simulink model "testemplanner_cs_old"  (R2020a)
settings: Solver=ode5  StartTime=0.0  StopTime=120  FixedStep=1/1000  RelTol=1e-3
PreLoadFcn:
  | mbxruntime.callbacks.PreLoadFcn(bdroot);
PostLoadFcn:
  | mbxruntime.callbacks.PostLoadFcn(bdroot);
InitFcn:
  | mbxruntime.callbacks.InitFcn(bdroot);
StartFcn:
  | mbxruntime.callbacks.StartFcn(bdroot);
StopFcn:
  | mbxruntime.callbacks.StopFcn(bdroot);
model workspace (MAT data in the model file):
  mbox_table : object (value not decoded)
  model_closed = 0
  sim_status = 0
values from neighbouring files (symbols this model uses):
  c_factor = 43.75    [emplanner_init.m]
  cf = -175016    [emplanner_init.m]
  cr = -130634    [emplanner_init.m]
  global_path_x = [0.057304 1.05668625507 2.05480936558 3.05165624935 4.04722112279 5.04150235808 6.03449985569 7.02621407764 8.01664569183 9.00579544113 9.99366409523 10.9802524329 ... (3001 elements, 3001x1)]    [global_path.mat]
  global_path_y = [8.29 8.29 8.29 8.29 8.29 8.29 8.29 8.29 8.29 8.29 8.29 8.29 ... (3001 elements, 3001x1)]    [global_path.mat]
  KD_PID_distance = 0.0    (= 0)    [emplanner_init.m]
  KD_PID_speed = 0    [emplanner_init.m]
  KI_PID_distance = 0.0    (= 0)    [emplanner_init.m]
  KI_PID_speed = 0    [emplanner_init.m]
  KP_PID_distance = 0.5    [emplanner_init.m]
  KP_PID_speed = 1.8    [emplanner_init.m]
  la = 1.265    [emplanner_init.m]
  lb = 2.947-1.265    (= 1.682)    [emplanner_init.m]
  LQR_K1 = k(:,1)'    [emplanner_init.m]
  LQR_K2 = k(:,2)'    [emplanner_init.m]
  LQR_K3 = k(:,3)'    [emplanner_init.m]
  LQR_K4 = k(:,4)'    [emplanner_init.m]
  m = 2020    [emplanner_init.m]
  rack_displacement = [-39.14 , -37.2 , -35.29 , -33.43 , -31.6 , -29.81 , -28.06 , -26.34 , -24.66 ,      -23.01 , -21.38 , -19.79 , -18.23 , -16.69 , -15.18 , -13.7 , -12.23 , -10.8 , -9.38 , -7.98 ,     -6.61 , -5.25 , -3.91 , -2.59 , -1.29 , 0 , 1.27 , 2.54 , 3.78 , 5.02 , 6.24 , 7.46 , 8.66 ,      9.86 , 11.05 , 12.24 , 13.41 , 14.59 , 15.76 , 16.92 , 18.09 , 19.25 , 20.42 , 21.59 , 22.76 ,      23.93 , 25.11 , 26 ...(+26 chars)    [emplanner_init.m]
  right_wheel_ground = [-70 ,-67.2 , -64.4 , -61.6 , -58.8 , -56 , -53.2 , -50.4 , -47.6 , -44.8 , -42 ,      -39.2 , -36.4 , -33.6 , -30.8 , -28 , -25.2 , -22.4 , -19.6 , -16.8 , -14 , -11.2 , -8.4 , -5.6 ,      -2.8 , 0 , 2.8 , 5.6 , 8.4 , 11.2 , 14 , 16.8 , 19.6 , 22.4 , 25.2 , 28 , 30.8 , 33.6 , 36.4 ,      39.2 , 42 , 44.8 , 47.6 , 50.4 , 53.2 , 56 , 58.8 , 61.6 , 64.4 , 67.2 , 70 ]    [emplanner_init.m]
  vx_break_point = zeros(1,5000)    [emplanner_init.m]
undefined symbols (not defined in the file or in its folder): aubr, DiscIntNeverNeededParam, tablebr, vubr
libraries: PreScanSimulinkLibrary x9, Solver_SF x1, simulink_extras x1
(part 5 of 6)

== matlab function testemplanner_cs_old/Audi_A8_Sedan_1/decision&planning module/EM_planner/calc plan start and stitch trajectory ==
  data: host_x input; plan_start_x output; host_y input; host_heading_xy input; host_vx input; host_vy input; host_ax input; host_ay input; pre_trajectory_x input; pre_trajectory_y input; pre_trajectory_heading input; pre_trajectory_kappa input; pre_trajectory_velocity input; pre_trajectory_accelerate input; pre_trajectory_time input; current_time input; plan_start_y output; plan_start_heading output; plan_start_kappa output; plan_start_vx output; plan_start_vy output; plan_start_ax output; plan_start_ay output; plan_start_time output; stitch_x output; stitch_y output; stitch_heading output; stitch_kappa output; stitch_velocity output; stitch_accelerate output; stitch_time output
function [plan_start_x,plan_start_y,plan_start_heading,plan_start_kappa,plan_start_vx,plan_start_vy,plan_start_ax,plan_start_ay,plan_start_time,stitch_x,stitch_y,...
    stitch_heading,stitch_kappa,stitch_velocity,stitch_accelerate,stitch_time] = fcn(host_x,host_y,host_heading_xy,host_vx,host_vy,host_ax,host_ay,pre_trajectory_x,pre_trajectory_y,...
    pre_trajectory_heading,pre_trajectory_kappa,pre_trajectory_velocity,pre_trajectory_accelerate,pre_trajectory_time,current_time)

%%作用：求得当前周期的规划起点，有两种方式，①一种方式是车辆当前位置与上一周期规划路径点相差较大，此时需要通过车辆动力学外推得到，②另一种方式是相差不大，直径将原有路径延长得到
%%输入：上一个周期规划出的路径的坐标点，航向，速度，加速度。车辆当前的坐标点、航向，速度，加速度，当前时间。
%%输出；规划起点的坐标点，航向，速度，加速度；待拼接轨迹的坐标点，航向，速度，加速度以及时间。

% 初始化待拼接轨迹，此轨迹主要用来进行拼接，加速计算过程，待拼接轨迹为计算的规划起点在原有轨迹上的位置向前取20个点，因此初始化一个20个点的数组
stitch_x=zeros(20,1)*nan;
stitch_y=zeros(20,1)*nan;
stitch_heading=zeros(20,1)*nan;
stitch_kappa=zeros(20,1)*nan;
stitch_velocity=zeros(20,1)*nan;
stitch_accelerate=zeros(20,1)*nan;
%时间初始化为-1，代表没有要拼接的轨迹
stitch_time=ones(20,1)*(-1);

%根据是否为第一次运行进行区分，
persistent is_first_run

if isempty(is_first_run)
    %算法首次运行，本来需要外推，但因为是首次运行就以车辆当前的位置作为规划起点
    is_first_run=0;
    plan_start_x=host_x;
    plan_start_y=host_y;
    plan_start_heading=host_heading_xy;
    plan_start_kappa=0;
    plan_start_vx=0;
    plan_start_vy=0;
    plan_start_ax=0;
    plan_start_ay=0;
    %规划起点时间戳为当前时间+100ms
    plan_start_time=current_time+0.1;
else
    %算法不是首次运行，可以正常运行
    
    %比较车辆当前实际位置与车辆规划位置的差别
    
    x_current=host_x;
    y_current=host_y;
    heading_current=host_heading_xy;
    kappa_current=0;%默认起点曲率为0
    %要转换为世界坐标系
    vx_current=host_vx*cos(heading_current)-host_vy*sin(heading_current);
    vy_current=host_vx*sin(heading_current)+host_vy*cos(heading_current);
    ax_current=host_ax*cos(heading_current)-host_ay*sin(heading_current);
    ay_current=host_ax*sin(heading_current)+host_ay*cos(heading_current);
    %接着遍历数组，求解根据规划，车辆当前应道在的位置
    for i=1:length(pre_trajectory_time)
        if(pre_trajectory_time(i)<=current_time)&&(pre_trajectory_time(i+1)>current_time)
           break; 
        else
        end
    end
    x_desire=pre_trajectory_x(i);
    y_desire=pre_trajectory_x(i);
    heading_desire=pre_trajectory_heading(i);
%     vx_desire=pre_trajectory_velocity*cos(pre_trajectory_heading(i));
%     vy_desire=pre_trajectory_velocity*sin(pre_trajectory_heading(i));
%     ax_desire=pre_trajectory_accelerate*cos(pre_trajectory_heading(i));
%     ay_desire=pre_trajectory_accelerate*sin(pre_trajectory_heading(i));
    
   %得到两个位置的误差
   %通过向量法计算误差
   %切向向量
   tor = [cos(heading_desire);sin(heading_desire)];
   %法向向量
   nor = [-sin(heading_desire);cos(heading_desire)];
   %两点向量
   error = [host_x;host_y]-[x_desire;y_desire];
   %纵向误差
   long_error = abs(error'*tor);
   %横向误差
   lat_error = abs(error'*nor);
   
   if (long_error>2.5)||(lat_error>0.5)   %控制误差过大，使用车辆动力学外推
        dt=0.1;
        plan_start_x=x_current+vx_current*dt+0.5*ax_current*dt*dt;
        plan_start_y=y_current+vy_current*dt+0.5*ay_current*dt*dt;
        plan_start_kappa=kappa_current;
        plan_start_vx=vx_current+ax_current*dt;
        plan_start_vy=vy_current+ay_current*dt;
        plan_start_ax=ax_current;
        plan_start_ay=ax_current;
        plan_start_heading=atan2(plan_start_vy,plan_start_vx);
    %规划起点时间戳为当前时间+100ms
        plan_start_time=current_time+0.1;
   else     %控制误差不大，则利用上一个周期规划路径找点
       for j=i:length(pre_trajectory_time)
            if (pre_trajectory_time(j)<=current_time+0.1)&&(pre_trajectory_time(j+1)>current_time+0.1)
                break;
            end
       end
        plan_start_x=pre_trajectory_x(j);
        plan_start_y=pre_trajectory_y(j);
        plan_start_heading=pre_trajectory_heading(j);
        plan_start_kappa=pre_trajectory_kappa(j);
        plan_start_vx=pre_trajectory_velocity(j)*cos(pre_trajectory_heading(j));
        plan_start_vy=pre_trajectory_velocity(j)*sin(pre_trajectory_heading(j));
        % 注意，由于是做圆周运动，所以加速度要先按照切向和法相进行分解
         %切向向量
         tor = [cos(heading_desire);sin(heading_desire)];
         %法向向量
         nor = [-sin(heading_desire);cos(heading_desire)];
        tor_a=pre_trajectory_accelerate(j)*tor;        %切向加速度
        nor_a=pre_trajectory_velocity(j)*pre_trajectory_kappa(j)*nor; %法向加速度=v^2/r
        %分别将切向加速度和法向加速度的x，y分量相加就是ax和ay
        plan_start_ax=tor_a(1)+nor_a(1);
        plan_start_ay=tor_a(2)+nor_a(2);
    %规划起点时间戳为当前时间+100ms
        plan_start_time=pre_trajectory_time(j); 
         %下面开始进行轨迹拼接
         %当前节点是j，如果j大于20，则往前拼接20个点，如果j<20，则能拼几个点就拼几个点。从stitch最后一个点开始拼，没有拼上的点time为-1
         if j>=21
             for k=j-1:-1:j-20
                 stitch_time(k)=pre_trajectory_time(k);
                 stitch_x(k)=pre_trajectory_x(k);
                 stitch_y(k)=pre_trajectory_y(k);
                 stitch_heading(k)=pre_trajectory_heading(k);
                 stitch_kappa(k)=pre_trajectory_kappa(k);
                 stitch_velocity(k) = pre_trajectory_velocity(k);
                 stitch_accelerate (k)= pre_trajectory_accelerate (k);
             end
         else
             for k=1:j-1
                 stitch_time(20+1-k)=pre_trajectory_time(j-k);
                 stitch_x(20+1-k)=pre_trajectory_x(j-k);
                 stitch_y(20+1-k)=pre_trajectory_y(j-k);
                 stitch_heading(20+1-k)=pre_trajectory_heading(j-k);
                 stitch_kappa(20+1-k)=pre_trajectory_kappa(j-k);
                 stitch_velocity(20+1-k) = pre_trajectory_velocity(j-k);
                 stitch_accelerate(20+1-k) = pre_trajectory_accelerate(j-k);
             end
         end
   end
   
   
   
end

== matlab function testemplanner_cs_old/Audi_A8_Sedan_1/decision&planning module/EM_planner/obs/Cart2Frenet/CalcSL2 ==
  data: frenet_l_set input; ax_set input; ay_set input; s_dot_set input; dl_set input; plan_start_proj_heading input; plan_start_proj_kappa input; s_dot2_set output; l_dot2_set output; ddl_set output
function [ s_dot2_set, l_dot2_set,ddl_set]=fcn(frenet_l_set,ax_set,ay_set,s_dot_set,dl_set,plan_start_proj_heading,plan_start_proj_kappa)
%作用：通过之前计算得到的l，s_dot、dl值以及已知的ax，ay值，计算s_dot2,l_dot2,以及ddl
 %首先做一个缓冲
 n=128;
 s_dot2_set=ones(n,1)*nan;
 l_dot2_set=ones(n,1)*nan;
 ddl_set=ones(n,1)*nan;

 for i=1:length(frenet_l_set)
     if isnan(frenet_l_set(i))
         break;
     end
    %先求自然坐标系的切向量和法向量
%切向量
tor=[cos(plan_start_proj_heading(i));sin(plan_start_proj_heading(i))];
%法向量
nor=[-sin(plan_start_proj_heading(i));cos(plan_start_proj_heading(i))];

ah=[ax_set(i);ay_set(i)];
l_dot2_set(i)=ah'*nor- plan_start_proj_kappa(i) * (1 - plan_start_proj_kappa(i) * frenet_l_set(i)) * s_dot_set(i)^2;
s_dot2_set(i)=(1/(1 - plan_start_proj_kappa(i) * frenet_l_set(i)))* (ah' * tor + 2 * plan_start_proj_kappa(i) * dl_set(i) * s_dot_set(i)^2);

if abs(s_dot2_set(i))<1e-6
    ddl_set(i)=0;
else
    ddl_set(i)=(l_dot2_set(i) - dl_set(i)*s_dot2_set(i))/(s_dot_set(i)^2);
 end
end

== matlab function testemplanner_cs_old/Audi_A8_Sedan_1/decision&planning module/EM_planner/obs/Cart2Frenet/Calcs_l_dot_dl ==
  data: frenet_l_set input; vx_set input; vy_set input; plan_start_proj_heading input; plan_start_proj_kappa input; s_dot_set output; l_dot_set output; dl_set output
function [ s_dot_set, l_dot_set,dl_set]=fcn(frenet_l_set,vx_set,vy_set,plan_start_proj_heading,plan_start_proj_kappa)
%作用：通过之前计算得到的s和l值以及计算的速度值，计算s_dot,l_dot,以及dl
 %首先做一个缓冲
 n=128;
 s_dot_set=ones(n,1)*nan;
 l_dot_set=ones(n,1)*nan;
 dl_set=ones(n,1)*nan;

 for i=1:length(frenet_l_set)
     if isnan(frenet_l_set(i))
         break;
     end
    %先求自然坐标系的切向量和法向量
%切向量
tor=[cos(plan_start_proj_heading(i));sin(plan_start_proj_heading(i))];
%法向量
nor=[-sin(plan_start_proj_heading(i));cos(plan_start_proj_heading(i))];

vh=[vx_set(i);vy_set(i)];
l_dot_set(i)=vh'*nor;
s_dot_set(i)=vh'*tor/(1-plan_start_proj_kappa(i)*frenet_l_set(i));

if abs(s_dot_set(i))<1e-6
    dl_set(i)=0;
else
    dl_set(i)=l_dot_set(i)/s_dot_set(i);
 end
end

== matlab function testemplanner_cs_old/Audi_A8_Sedan_1/decision&planning module/EM_planner/DP path ==
  data: plan_start_s input; dp_path_s_init output; plan_start_l input; plan_start_dl input; plan_start_ddl input; obs_s_set input; obs_l_set input; w_smooth_dl_cost input; w_collision_cost input; w_ref_cost input; w_smooth_ddl_cost input; w_smooth_dddl_cost input; col input; row input; sample_s input; sample_l input; dp_path_l_init output
function [dp_path_s_init,dp_path_l_init] = fcn(plan_start_s,plan_start_l,plan_start_dl,plan_start_ddl,obs_s_set,obs_l_set,w_smooth_dl_cost,w_collision_cost,w_ref_cost,w_smooth_ddl_cost,w_smooth_dddl_cost,col,row,sample_s,sample_l)
%%作用：撒点，通过动态规划算出代价最小的路径点集合，算出要进行优化的凸空间
%%输入：规划起点的s，l,dl,ddl,静态障碍物的s，l集合，dl，ddl，dddl平滑代价，参考线代价以及碰撞代价权重
%%行数：为奇数，列数；采样的横向距离以及纵向距离

%%输出：计算得到的路径点s，l初始值

%首先定义一个代价数组，代表从起点到当前i，j点的总代价，均初始化为inf无穷大
node=ones(col,row)*inf;

%再定义一个pre_node,用来表征node的父节点的坐标索引，均初始化为0，0；假设所有节点的父节点均为起点

pre_node=zeros(col,row);
%首先计算第一列的点的cost，调用CalccostFromStart函数进行计算
for i=1:row
    node(1,i)=CalccostFromStart(plan_start_s,plan_start_l,plan_start_dl,plan_start_ddl,obs_s_set,obs_l_set,w_smooth_dl_cost,w_collision_cost,w_ref_cost,w_smooth_ddl_cost,w_smooth_dddl_cost,i,row,sample_s,sample_l);
end
%计算从第二列开始的每一列的最小代价值以及其父节点的索引值，调用CalccostFromNeibor函数进行计算
for j=2:col
    for k =1:row
    [node,pre_node]=CalccostFromNeibor(plan_start_s,node,pre_node,k,j,obs_s_set,obs_l_set,w_smooth_dl_cost,w_collision_cost,w_ref_cost,w_smooth_ddl_cost,w_smooth_dddl_cost,row,sample_s,sample_l);
    end
end
% 找到最后一列中代价最小的节点
min_cost=node(1,end);
index=1;
for i=2:row
    min_cost_temp=node(i,end);
    if min_cost_temp<min_cost
        index=i;
        min_cost=min_cost_temp;
    else
    end
end

%因为不知道有多少个点，所以做一个缓冲
dp_path_s_init=ones(15,1)* -1;
dp_path_l_init=ones(15,1)* -1;

temp_node=zeros(15,1);

%从最后一个节点开始，反向找到最小代价路径上的所有点，并放入集合中
for i=col:-1:1
    
    temp_node(i)=pre_node(index,i);
    index=pre_node(index,i);
end
%确定路径上点的s，l值
for i=1:col
dp_path_s_init(i)=sample_s*i;
dp_path_l_init(i)=sample_l*(temp_node(col+1-i)-(row+1)/2);
end
end

%函数CalccostFromNeibor，计算从上一列的临近点到这个点的最小cost值和其父节点的行索引
function [node,pre_node]=CalccostFromNeibor(plan_start_s,node,pre_node,k,j,obs_s_set,obs_l_set,w_smooth_dl_cost,w_collision_cost,w_ref_cost,w_smooth_ddl_cost,w_smooth_dddl_cost,row,sample_s,sample_l)
% %作用： 计算从从上一列的临近点到这个点的最小cost值和其父节点的行索引
  %输入：起点的s，l，障碍物的s,l,dl,ddl,dddl平滑权重，障碍物碰撞权重，参考线权重，当前所在行数，列数，总行数，采样s，l，node和pre_node数组
  %输出：更新后的node和pre_node数组
  %dl，ddl设为0，因为DP仅仅是为了粗略开辟凸空间，不用太精细。
start_s=plan_start_s+sample_s*(j-1);
end_s=start_s+plan_start_s+sample_s*(j);
start_dl=0;
start_ddl=0;
end_dl=0;
end_ddl=0;
cost=zeros(row,1);
%确定起点和终点参数，计算五次多项式系数
for i=1:row
start_l=sample_l*(i-(row+1)/2);
end_l=sample_l*(k-(row+1)/2);
%调用函数计算五次多项式系数
coffee=Calccoffee(start_s,start_l,start_dl,start_ddl,end_s,end_l,end_dl,end_ddl);

s_set=zeros(10,1);
l_set=zeros(10,1);
dl_set=zeros(10,1);
ddl_set=zeros(10,1);
dddl_set=zeros(10,1);

%找10个点进行代价计算
for n=1:10
    s_set(n)=start_s+sample_s/10*(n-1);
    l_set(n)=coffee(1)*(s_set(n))^5+coffee(2)*(s_set(n))^4+coffee(3)*(s_set(n))^3+coffee(4)*(s_set(n))^2+coffee(5)*(s_set(n))+coffee(6);
    dl_set(n)=5*coffee(1)*(s_set(n))^4+4*coffee(2)*(s_set(n))^3+3*coffee(3)*(s_set(n))^2+2*coffee(4)*(s_set(n))+coffee(5);
    ddl_set(n)=20*coffee(1)*(s_set(n))^3+12*coffee(2)*(s_set(n))^2+6*coffee(3)*(s_set(n))+2*coffee(4);
    dddl_set(n)=60*coffee(1)*(s_set(n))^2+24*coffee(2)*(s_set(n))+6*coffee(3);
end
%首先计算平滑带代价和参考线代价
smooth_cost=w_smooth_dl_cost*(dl_set'*dl_set)+w_smooth_ddl_cost*(ddl_set'*ddl_set)+w_smooth_dddl_cost*(dddl_set'*dddl_set);
ref_cost=w_ref_cost*(l_set'*l_set);
%接着计算障碍物代价
collision_cost=0;
for m=1:length(obs_s_set)
    if isnan(obs_s_set(m))
        break;
    end
    s_err=obs_s_set(m)*ones(10,1)-s_set;
    l_err=obs_l_set(m)*ones(10,1)-l_set;
    err_squard=s_err.^2+l_err.^2;
    %调用障碍物代价模型函数CalcObsCost进行计算
    collision_cost_one=CalcObsCost(err_squard,w_collision_cost);
    collision_cost=collision_cost+collision_cost_one;
end

cost(i)=smooth_cost+ref_cost+collision_cost+node(i,j-1);
end
index=1;
min_cost=cost(1);
for h =2:row
   
    min_cost_temp=cost(h);
    if min_cost_temp<min_cost
        index=h;
        min_cost=min_cost_temp;
    else
    end
end
 pre_node(k,j)=index;
 node(k,j)=min_cost;
end




%函数CalccostFromStart，计算从起点到第一列的点的cost值
function cost=CalccostFromStart(plan_start_s,plan_start_l,plan_start_dl,plan_start_ddl,obs_s_set,obs_l_set,w_smooth_dl_cost,w_collision_cost,w_ref_cost,w_smooth_ddl_cost,w_smooth_dddl_cost,node_row,row,sample_s,sample_l)

  %作用： 计算从起点到第一列的点的cost值
  %输入：起点的s，l，dl，ddl,障碍物的s,l,dl,ddl,dddl平滑权重，障碍物碰撞权重，参考线权重，当前所在行数，总行数，采样s，l
  %输出：代价和
start_s=plan_start_s;
start_l=plan_start_l;
start_dl=plan_start_dl;
start_ddl=plan_start_ddl;
end_s=start_s+sample_s;
end_l=sample_l*(node_row-(row+1)/2);
end_dl=0;
end_ddl=0;
%调用函数计算五次多项式系数
coffee=Calccoffee(start_s,start_l,start_dl,start_ddl,end_s,end_l,end_dl,end_ddl);

s_set=zeros(10,1);
l_set=zeros(10,1);
dl_set=zeros(10,1);
ddl_set=zeros(10,1);
dddl_set=zeros(10,1);

%找10个点进行代价计算
for i=1:10
    s_set(i)=start_s+sample_s/10*(i-1);
    l_set(i)=coffee(1)*(s_set(i))^5+coffee(2)*(s_set(i))^4+coffee(3)*(s_set(i))^3+coffee(4)*(s_set(i))^2+coffee(5)*(s_set(i))+coffee(6);
    dl_set(i)=5*coffee(1)*(s_set(i))^4+4*coffee(2)*(s_set(i))^3+3*coffee(3)*(s_set(i))^2+2*coffee(4)*(s_set(i))+coffee(5);
    ddl_set(i)=20*coffee(1)*(s_set(i))^3+12*coffee(2)*(s_set(i))^2+6*coffee(3)*(s_set(i))+2*coffee(4);
    dddl_set(i)=60*coffee(1)*(s_set(i))^2+24*coffee(2)*(s_set(i))+6*coffee(3);
end
%首先计算平滑带代价和参考线代价
smooth_cost=w_smooth_dl_cost*(dl_set'*dl_set)+w_smooth_ddl_cost*(ddl_set'*ddl_set)+w_smooth_dddl_cost*(dddl_set'*dddl_set);
ref_cost=w_ref_cost*(l_set'*l_set);
%接着计算障碍物代价
collision_cost=0;
for i=1:length(obs_s_set)
    if isnan(obs_s_set(i))
        break;
    end
    s_err=obs_s_set(i)*ones(10,1)-s_set;
    l_err=obs_l_set(i)*ones(10,1)-l_set;
    err_squard=s_err.^2+l_err.^2;
     %调用障碍物代价模型函数CalcObsCost进行计算
    collision_cost_one=CalcObsCost(err_squard,w_collision_cost);
    collision_cost=collision_cost+collision_cost_one;
end

cost=smooth_cost+ref_cost+collision_cost;


end
function coffee=Calccoffee(start_s,start_l,start_dl,start_ddl,end_s,end_l,end_dl,end_ddl)
  %作用：计算五次多项式系数
  %输入：起点和终点的s,l,dl,ddl共6个值
  %输出：六个权重系数
    start_s2=start_s*start_s;
    start_s3=start_s2*start_s;
    start_s4=start_s3*start_s;
    start_s5=start_s4*start_s;
    end_s2=end_s*end_s;
    end_s3=end_s2*end_s;
    end_s4=end_s3*end_s;
    end_s5=end_s4*end_s;
    A=[1,start_s,start_s2,start_s3,start_s4,start_s5;
       0,1,2*start_s,3*start_s2,4*start_s3,5*start_s4;
       0,0,2,6*start_s,12*start_s2,20*start_s3;
       1,end_s,end_s2,end_s3,end_s4,end_s5;
       0,1,2*end_s,3*end_s2,4*end_s3,5*end_s4;
        0,0,2,6*end_s,12*end_s2,20*end_s3;];
    B=[start_l;start_dl;start_ddl;end_l;end_dl;end_ddl];
    coffee=A\B;
end
function obscost=CalcObsCost(err_squard,w_collision_cost)
  %作用： %建立一个障碍物评估模型，进行代价评估
  %输入：与障碍物的横纵向距离平方和，碰撞权重
  %输出：障碍物代价和
    cost=0;
    for i=1:length(err_squard)
        if err_squard(i)>16
        elseif err_squard(i)<=16 &&err_squard(i)>=9
            cost=cost+1000/err_squard(i);
        else
            cost=cost+w_collision_cost;
        end
    end
    obscost=cost;
end

== matlab function testemplanner_cs_old/Audi_A8_Sedan_1/decision&planning module/EM_planner/DP node generate ==
  data: dp_path_s_init input; dp_path_s_final output; dp_path_l_init input; plan_start_s input; plan_start_l input; plan_start_dl input; plan_start_ddl input; dp_path_l_final output; dp_path_dl_final output; dp_path_ddl_final output
function [dp_path_s_final,dp_path_l_final,dp_path_dl_final,dp_path_ddl_final] = fcn(dp_path_s_init,dp_path_l_init,plan_start_s,plan_start_l,plan_start_dl,plan_start_ddl)
%%作用：对DP求得的路径进行路径点加密
%%输入：dp求得的点s，l参数，规划起点的s，l，dl，ddl参数
%%输出：加密后的路径点的s，l，dl，ddl参数
%每隔1m取一个点
ds=1;
%初始化输出数组
dp_path_s_final=ones(60,1)*nan;
dp_path_l_final=ones(60,1)*nan;
dp_path_dl_final=ones(60,1)*nan;
dp_path_ddl_final=ones(60,1)*nan;

%初始化过程变量
cur_node_s=0;
l_temp=[];
dl_temp=[];
ddl_temp=[];
%初始化路径起点
start_s=plan_start_s;
start_l=plan_start_l;
start_dl=plan_start_dl;
start_ddl=plan_start_ddl;
%遍历整个输入的s集合，进行节点加密
for i=1:length(dp_path_s_init)
    if dp_path_s_init==-1
        break;
    end
    end_s=dp_path_s_init(i);
    end_l=dp_path_l_init(i);
    end_dl=0;
    end_ddl=0;
    coffee=Calccoffee(start_s,start_l,start_dl,start_ddl,end_s,end_l,end_dl,end_ddl);
    for j=1:10000
        if(start_s+ds*(j-1))<end_s
            cur_node_s=start_s+ds*(j-1);
            l_cur=coffee(1)*(cur_node_s)^5+coffee(2)*(cur_node_s)^4+coffee(3)*(cur_node_s)^3+coffee(4)*(cur_node_s)^2+coffee(5)*(cur_node_s)+coffee(6);
            dl_cur=5*coffee(1)*(cur_node_s)^4+4*coffee(2)*(cur_node_s)^3+3*coffee(3)*(cur_node_s)^2+2*coffee(4)*(cur_node_s)+coffee(5);
            ddl_cur=20*coffee(1)*(cur_node_s)^3+12*coffee(2)*(cur_node_s)^2+6*coffee(3)*(cur_node_s)+2*coffee(4);
            l_temp=[l_temp,l_cur];
            dl_temp=[dl_temp,dl_cur];
            ddl_temp=[ddl_temp,ddl_cur];
            
        else
            break;
        end
    end
      start_s=end_s;
      start_l=end_l;
      start_dl=end_dl;
      start_ddl=end_ddl;
end

for k=1:length(l_temp)
    if k==61
        break;
    else
        dp_path_s_final(k)=plan_start_s+ds*(k-1);
        dp_path_l_final(k)=l_temp(k);
        dp_path_dl_final(k)=dl_temp(k);
        dp_path_ddl_final(k)=ddl_temp(k);
    end
end

end

function coffee=Calccoffee(start_s,start_l,start_dl,start_ddl,end_s,end_l,end_dl,end_ddl)
  %作用：计算五次多项式系数
  %输入：起点和终点的s,l,dl,ddl共6个值
  %输出：六个权重系数
    start_s2=start_s*start_s;
    start_s3=start_s2*start_s;
    start_s4=start_s3*start_s;
    start_s5=start_s4*start_s;
    end_s2=end_s*end_s;
    end_s3=end_s2*end_s;
    end_s4=end_s3*end_s;
    end_s5=end_s4*end_s;
    A=[1,start_s,start_s2,start_s3,start_s4,start_s5;
       0,1,2*start_s,3*start_s2,4*start_s3,5*start_s4;
       0,0,2,6*start_s,12*start_s2,20*start_s3;
       1,end_s,end_s2,end_s3,end_s4,end_s5;
       0,1,2*end_s,3*end_s2,4*end_s3,5*end_s4;
        0,0,2,6*end_s,12*end_s2,20*end_s3;];
    B=[start_l;start_dl;start_ddl;end_l;end_dl;end_ddl];
    coffee=A\B;
end

== matlab function testemplanner_cs_old/Audi_A8_Sedan_1/decision&planning module/EM_planner/increase st point count ==
  data: s_init input; s output; s_dot_init input; s_dot2_init input; relative_time_init input; s_dot output; s_dot2 output; relative_time output
function [s,s_dot,s_dot2,relative_time] = fcn(s_init,s_dot_init,s_dot2_init,relative_time_init)
%该函数将增密s s_dot s_dot2
% 为什么需要增密，因为控制的执行频率是规划的10倍，轨迹点如果不够密，必然会导致规划效果不好
% 但是若在速度二次规划中点取的太多，会导致二次规划的矩阵规模太大计算太慢
% 所以方法是在二次规划中选取少量的点优化完毕后，在用此函数增密
T = relative_time_init(end);
n = 401;
dt = T/(n-1);
s = zeros(n,1);
s_dot = zeros(n,1);
s_dot2 = zeros(n,1);
relative_time = zeros(n,1);
for i = 1:n
    current_t = (i-1)*dt;
    for j = 1:length(relative_time_init)-1
        if relative_time_init(j) <= current_t && relative_time_init(j+1) > current_t
            break;
        end
    end
    x = current_t - relative_time_init(j);
    s(i) = s_init(j) + s_dot_init(j)*x + (1/3)*s_dot2_init(j)*x^2 + (1/6)*s_dot2_init(j+1)*x^2; 
    s_dot(i) = s_dot_init(j) + 0.5*s_dot2_init(j)*x + 0.5*s_dot2_init(j+1)*x;
    s_dot2(i) = s_dot2_init(j) + (s_dot2_init(j+1) - s_dot2_init(j))*x/(relative_time_init(j+1) - relative_time_init(j));
    relative_time(i) = current_t;
end

== matlab function testemplanner_cs_old/Audi_A8_Sedan_1/decision&planning module/EM_planner/Frenet2Cart ==
  data: s_set input; x_set output; l_set input; dl_set input; ddl_set input; frenet_s input; frenet_l input; frenet_heading input; frenet_kappa input; index2s input; y_set output; heading_set output; kappa_set output
function [x_set,y_set,heading_set,kappa_set] = fcn(s_set,l_set,dl_set,ddl_set,frenet_s,frenet_l,frenet_heading,frenet_kappa,index2s)

%%作用：实现frenet坐标转换为笛卡尔坐标，进行控制.整个流程是先根据s求匹配点的x,y，再根据ds求投影点的x，y,再根据dl求要转换点的x,y
%%输入：frenet坐标下路径的s，l,dl,ddl;参考线的s,l,heading,kappa以及index2s

%%输出：路径在笛卡尔坐标系下的x,y,heading,kappa

%不知道要转换多少个点，因此进行缓冲

n=128;
%初始化输出
x_set=ones(n,1)*nan;
y_set=ones(n,1)*nan;
heading_set=ones(n,1)*nan;
kappa_set=ones(n,1)*nan;
for i=1:length(s_set)
    if isnan(s_set(i))
        break;
    end
    %写一个函数，用来计算路径s,l所对应的投影点的直角坐标系x，y，heading，kappa
    [proj_x,proj_y,proj_heading,proj_kappa]=calcProjPoint(s_set(i),frenet_s,frenet_l,frenet_heading,frenet_kappa,index2s);
    nor=[-sin(proj_heading);cos(proj_heading)];
    point_cert=[proj_x;proj_y]+l_set(i)*nor;
    x_set(i)=point_cert(1);
    y_set(i)=point_cert(2);
    heading_set(i) = proj_heading + atan(dl_set(i)/(1 - proj_kappa * l_set(i)));
    % 近似认为 kappa' == 0,frenet转cartesian公式，见第一章第三节评论区的链接
    kappa_set(i) = ((ddl_set(i) + proj_kappa * dl_set(i) * tan(heading_set(i) - proj_heading)) * ...
        (cos(heading_set(i) - proj_heading)^2)/(1 - proj_kappa * l_set(i)) + proj_kappa) * ...
        cos(heading_set(i) - proj_heading)/(1 - proj_kappa * l_set(i));
    
end
end


function  [proj_x,proj_y,proj_heading,proj_kappa]=calcProjPoint(s,frenet_x,frenet_y,frenet_heading,frenet_kappa,index2s)
   match_point_index=0;
    for j=1:length(index2s)
        if index2s(j)<s
            match_point_index=j+1;
        else
            break;
        end
    end
    ds=s-index2s(match_point_index);
    tor=[cos(frenet_heading(match_point_index));sin(frenet_heading(match_point_index))];
    point=[frenet_x((match_point_index));frenet_y((match_point_index))]+ds*tor;
    proj_x=point(1);
    proj_y=point(2);
    proj_heading=frenet_heading((match_point_index))+ds*frenet_kappa(match_point_index);
    proj_kappa=frenet_kappa(match_point_index);
    end

== matlab function testemplanner_cs_old/Audi_A8_Sedan_1/decision&planning module/EM_planner/stitch trajectory ==
  data: trajectory_x input; trajectory_x_final output; trajectory_y input; trajectory_heading input; trajectory_kappa input; trajectory_speed input; trajectory_accel input; trajectory_time input; stitch_x input; stitch_y input; stitch_heading input; stitch_kappa input; stitch_speed input; stitch_accel input; stitch_time input; trajectory_y_final output; trajectory_heading_final output; trajectory_kappa_final output; trajectory_speed_final output; trajectory_accel_final output; trajectory_time_final output
function [trajectory_x_final,trajectory_y_final,trajectory_heading_final,trajectory_kappa_final,trajectory_speed_final,trajectory_accel_final,trajectory_time_final] = fcn(trajectory_x,trajectory_y,trajectory_heading,trajectory_kappa,trajectory_speed,trajectory_accel,trajectory_time,...
    stitch_x,stitch_y,stitch_heading,stitch_kappa,stitch_speed,stitch_accel,stitch_time)

n=401+20;

trajectory_x_final=zeros(n,1);
trajectory_y_final=zeros(n,1);
trajectory_heading_final=zeros(n,1);
trajectory_kappa_final=zeros(n,1);
trajectory_speed_final=zeros(n,1);
trajectory_accel_final=zeros(n,1);
trajectory_time_final=zeros(n,1);



trajectory_x_final=[stitch_x;trajectory_x];
trajectory_y_final=[stitch_y;trajectory_y];
trajectory_heading_final=[stitch_heading;trajectory_heading];
trajectory_kappa_final=[stitch_kappa;trajectory_kappa];
trajectory_speed_final=[stitch_speed;trajectory_speed];
trajectory_accel_final=[stitch_accel;trajectory_accel];
trajectory_time_final=[stitch_time;trajectory_time];
end

== matlab function testemplanner_cs_old/Audi_A8_Sedan_1/control module1/MATLAB Function ==
  data: trajectory_x_final input; x_r output; trajectory_y_final input; trajectory_heading_final input; trajectory_kappa_final input; trajectory_speed_final input; trajectory_accel_final input; trajectory_time_final input; current_time input; y_r output; theta_r output; kappa_r output; speed output; accel output; control_predict_time input
function [x_r,y_r,theta_r,kappa_r,speed,accel] = fcn(trajectory_x_final,trajectory_y_final,trajectory_heading_final,trajectory_kappa_final,trajectory_speed_final,...
    trajectory_accel_final,trajectory_time_final,current_time,control_predict_time)

%%作用，根据当前时间，选取轨迹点集合上合适的点进行插值，生成控制用的x，y,heading,kappa,speed,acc

%%输入：轨迹点集合的x，y,heading,kappa,acc,时间戳，当前时间。

%%输出：控制点用的x，y,heading,kappa,speed,acc


%首先控制也要进行预瞄,时间是0.01/0.02
control_time=current_time+control_predict_time;
start_index=1;
%%为了防止轨迹所对应的时间戳不可信（时间戳为-1），找到可用的起点
while trajectory_time_final(start_index)==-1
        start_index=start_index+1;
end

%%正常来讲可以通过插值的方式（调用matlab函数interp1）来计算控制点对应的插值
%%但是存在着两种异常工况需要进行处理
%%①interp1在段点插值会得到nan
%%②interp1要求x轴的数必须单调递增

%%在起步时：在t=0~100ms时刻，规划还未完成，无轨迹信息，也就是说轨迹的时间都是0，而控制每10ms执行异常，因此此时给控制的轨迹信息应该全为起点的信息
%%保证车辆不动

if trajectory_time_final(start_index)~=0 &&control_time>trajectory_time_final(start_index) %%正常运行分支
    x_r=interp1(trajectory_x_final(start_index:end),trajectory_time_final(start_index:end),control_time);
    y_r=interp1(trajectory_y_final(start_index:end),trajectory_time_final(start_index:end),control_time);
    theta_r=interp1(trajectory_heading_final(start_index:end),trajectory_time_final(start_index:end),control_time);
    if theta_r==-pi
        theta_r=pi;
    elseif theta_r==2*pi||theta_r==-2*pi
        theta_r=0;
    else
    end
    
    kappa_r=interp1(trajectory_kappa_final(start_index:end),trajectory_time_final(start_index:end),control_time);
    speed=interp1(trajectory_speed_final(start_index:end),trajectory_time_final(start_index:end),control_time);
    accel=interp1(trajectory_accel_final(start_index:end),trajectory_time_final(start_index:end),control_time);
else
    
    x_r=trajectory_x_final(start_index);
    y_r=trajectory_y_final(start_index);
    theta_r=trajectory_heading_final(start_index);
    kappa_r=trajectory_kappa_final(start_index);
    speed=trajectory_speed_final(start_index);
    accel=trajectory_accel_final(start_index);

end

end

== matlab function testemplanner_cs_old/Audi_A8_Sedan_1/decision&planning module/EM_planner/calc path length and map between point and s ==
  data: trajectory_x input; path_s_end output; trajectory_y input; path_s output
function [path_s_end,path_s] = fcn(trajectory_x,trajectory_y)
% 该函数将计算以trajectory的s 与 x y 的对应关系，可以看作是trajectory index2s
n = length(trajectory_x);
path_s = zeros(n,1);
sum = 0;
for i = 2:length(trajectory_x)
    if isnan(trajectory_x(i))
        break;
    end
    sum = sum + sqrt((trajectory_x(i) - trajectory_x(i-1))^2 + (trajectory_y(i) - trajectory_y(i-1))^2);
    path_s(i) = sum;
end
% 计算出trajectory的长度
if i == n
    path_s_end = path_s(end);
else
    % 因为循环的退出条件为isnan(trajectory_x(i)) 所以 i 所对应的数为 nan 
    path_s_end = path_s(i - 1);
end

== matlab function testemplanner_cs_old/Audi_A8_Sedan_1/decision&planning module/EM_planner/path and speed merge ==
  data: s input; trajectory_x output; s_dot input; s_dot2 input; relative_time input; current_time input; path_s input; trajectory_x_init input; trajectory_y_init input; trajectory_heading_init input; trajectory_kappa_init input; trajectory_y output; trajectory_heading output; trajectory_kappa output; trajectory_speed output; trajectory_accel output; trajectory_time output
function [trajectory_x,trajectory_y,trajectory_heading,trajectory_kappa,trajectory_speed,trajectory_accel,trajectory_time] = ...
    fcn(s,s_dot,s_dot2,relative_time,current_time,path_s,trajectory_x_init,trajectory_y_init,trajectory_heading_init,trajectory_kappa_init)
% 该函数将合并path和speed
% 由于path 是 60个点，speed 有 401个点，合并后，path和speed有401个点，因此需要做插值
n = 401;
trajectory_x = zeros(n,1);
trajectory_y = zeros(n,1);
trajectory_heading = zeros(n,1);
trajectory_kappa = zeros(n,1);
trajectory_speed = zeros(n,1);

trajectory_accel = zeros(n,1);
index = 1;
% 由于trajectory_x_init中不是所有的值都有效，(有nan) 所以要找到有效值的范围
while ~isnan(trajectory_x_init(index)) 
    index = index + 1;
end
index = index - 1;
trajectory_time = zeros(n,1);
for i = 1:n-1
    %interp1 线性插值
    % 若 x = [1,2] y = [3,4]
    %interp1(x,y,1.5) 会得到3.5
    %interp1 的缺点是 在端点或超过端点的，结果为nan
    % interp1(x,y,2) 不会等于4 而是会等于nan
    % interp1(x,y,6) 也会等于nan，所以在端点处要单独处理
    trajectory_x(i) = interp1(path_s(1:index),trajectory_x_init(1:index),s(i));
    trajectory_y(i) = interp1(path_s(1:index),trajectory_y_init(1:index),s(i));
    trajectory_heading(i) = interp1(path_s(1:index),trajectory_heading_init(1:index),s(i));
    trajectory_kappa(i) = interp1(path_s(1:index),trajectory_kappa_init(1:index),s(i));
    trajectory_time(i) = relative_time(i) + current_time;%速度规划会得到相对时间，转换成绝对时间
    trajectory_speed(i) = s_dot(i);
    trajectory_accel(i) = s_dot2(i);
end
% 端点单独处理
trajectory_x(end) = trajectory_x_init(end);
trajectory_y(end) = trajectory_y_init(end);
trajectory_heading(end) = trajectory_heading_init(end);
trajectory_kappa(end) = trajectory_kappa_init(end);
trajectory_time(end) = relative_time(end) + current_time;
trajectory_speed(end) = s_dot(end);
trajectory_accel(end) = s_dot2(end);

== stateflow chart testemplanner_cs_old/Audi_A8_Sedan_1/Schedule OS ==
  (default) -> (junction 5)
  (junction 5) -> (junction 9) [order 1] : [i>100]
  (junction 5) -> (junction 10) [order 2] : {i = i+1;}
  (junction 9) -> (junction 12) : {
      | do_planning;
      | i = 0;
      | }
  (junction 12) -> (junction 10)
  (junction 10) -> (junction 15)
  (junction 15) -> (junction 17) [order 1] : [j>10]
  (junction 15) -> (junction 21) [order 2] : {j = j+1}
  (junction 17) -> (junction 19) : {
      | do_control;
      | j = 0;
      | }
  (junction 19) -> (junction 21)
  (junction 21) -> (junction 24)
  data: i local =1; j local =1
  events: do_planning output FUNCTION_CALL_EVENT; do_control output FUNCTION_CALL_EVENT

== matlab function testemplanner_cs_old/Audi_A8_Sedan_1/decision&planning module/EM_planner/calc speed planning start condition ==
  data: plan_start_vx input; plan_start_s_dot output; plan_start_vy input; plan_start_ax input; plan_start_ay input; plan_start_heading input; plan_start_s_dot2 output
function [plan_start_s_dot,plan_start_s_dot2] = fcn(plan_start_vx,plan_start_vy,plan_start_ax,plan_start_ay,plan_start_heading)
% 该函数计算速度规划的初始条件
tor = [cos(plan_start_heading);sin(plan_start_heading)];
v_t = tor'*[plan_start_vx;plan_start_vy];
a_t = tor'*[plan_start_ax;plan_start_ay];
plan_start_s_dot = v_t;
plan_start_s_dot2 = a_t;

== matlab function testemplanner_cs_old/Audi_A8_Sedan_1/decision&planning module/EM_planner/simple speed qp planning ==
  data: plan_start_s_dot input; s_init output; plan_start_s_dot2 input; s_end input; recommend_T input; s_dot_init output; s_dot2_init output; relative_time_init output
function [s_init,s_dot_init,s_dot2_init,relative_time_init] = fcn(plan_start_s_dot,plan_start_s_dot2,s_end,recommend_T)
%简单速度二次规划
coder.extrinsic("quadprog")
n = 51;
s_init = zeros(n,1);
s_dot_init = zeros(n,1);
s_dot2_init = zeros(n,1);
relative_time_init = zeros(n,1);

Aeq = zeros(3*n,2*n - 2);
beq = zeros(2*n - 2,1);
lb = ones(3*n,1);
ub = lb;
dt = recommend_T/(n-1);
A_sub =[1,0;
        dt,1;
        (1/3)*dt^2,(1/2)*dt;
        -1,0;
        0,-1;
        (1/6)*dt^2,dt/2];
for i = 1:n - 1
    Aeq(3*i-2:3*i+3,2*i-1:2*i) = A_sub;
end

for i = 1:n
   lb(3*i - 2) = -inf;
   lb(3*i - 1) = 0;
   lb(3*i) = -8;
   ub(3*i - 2) = inf;
   ub(3*i - 1) = 50;
   ub(3*i) = 2;
end
lb(1) = 0;
lb(2) = plan_start_s_dot;
lb(3) = plan_start_s_dot2;
ub(1) = lb(1);
ub(2) = lb(2);
ub(3) = lb(3);
lb(3*n - 2) = s_end;
ub(3*n - 2) = s_end;
A3 = zeros(3*n,3*n);
A4 = zeros(3*n,n - 1);
A4_sub =[0;0;1;0;0;-1];
for i = 1:n - 1
   A3(3*i,3*i) = 1;
   A4(3*i-2:3*i+3,i:i) = A4_sub;
end
A3(3*n,3*n) = 1;
H = A3 + 100*(A4*A4');
H = 2*H;
f = zeros(3*n,1);
X = quadprog(H,f,[],[],Aeq',beq,lb,ub);
for i = 1:n
   s_init(i) = X(3*i - 2);
   s_dot_init(i) = X(3*i - 1);
   s_dot2_init(i) = X(3*i);
   relative_time_init(i) = (i - 1)*dt;
end

== matlab function testemplanner_cs_old/Audi_A8_Sedan_1/decision&planning module/referenceline provider/MATLAB Function2 ==
  data: path_x input; path_heading output; path_y input; path_kappa output
function [path_heading,path_kappa] = fcn(path_x,path_y)
%%通过全局轨迹点坐标求解轨迹点的航向以及曲率
%输入：坐标点的x,y坐标
%输出：坐标点与x轴夹角航向以及此点的曲率大小
%原理：
%    dheading=atan（dy/dx）
%    dw=dheading/ds
%    ds=sqrt((dx^2+dy^2))
%求航向角时使用atan函数会涉及角的多值性，因此使用四象限atan函数和中点欧拉法求解
dx=diff(path_x);
dy = diff(path_y);
dx_pre=[dx(1);dx];
dx_after=[dx;dx(end)];
dy_pre=[dy(1);dy];
dy_after=[dy;dy(end)];
dx_final=(dx_after+dx_pre)/2;
dy_final=(dy_after+dy_pre)/2;
ds=sqrt(dx_final.^2+dy_final.^2);
d_heading=atan2(dy_final,dx_final);
diff_d_heading=diff(d_heading);
d_heading_pre=[diff_d_heading(1);diff_d_heading];
d_heading_after=[diff_d_heading;diff_d_heading(end)];
d_heading_final=(d_heading_pre+d_heading_after)/2;
dw=sin(d_heading_final)./ds;%使用sin(a)=a,当a非常小时


path_heading=d_heading_final;
path_kappa=dw;

== matlab function testemplanner_cs_old/Audi_A8_Sedan_1/decision&planning module/referenceline provider/general fast algorithm to find projection point info1 ==
  data: x_set input; match_point_index_set output; y_set input; path_x input; path_y input; proj_x_set output; proj_y_set output; proj_heading_set output; proj_kappa_set output; path_heading input; path_kappa input
% function [match_point_index_set,proj_x_set,proj_y_set,proj_heading_set,proj_kappa_set] = fcn(x_set,y_set,path_x,path_y,path_heading,path_kappa)
% %该函数是一个通用函数，找到x_set,y_set在path_x,path_y的匹配点的编号，以及投影点在直角坐标系下的(x,y,theta,kappa)
% %最多可以处理128个点
% 
% match_point_index_set = ones(128,1)*nan;
% proj_x_set = ones(128,1)*nan;
% proj_y_set = ones(128,1)*nan;
% proj_heading_set = ones(128,1)*nan;
% proj_kappa_set = ones(128,1)*nan;
% 
% 
% persistent is_first_run;
% persistent init_search_index_set;
% if isempty(is_first_run)
%     is_first_run = 0; 
%     init_search_index_set = ones(128,1)*nan;
%     for i = 1:length(x_set)
%         if isnan(x_set(i))
%             break;
%         else
%             increase_count = 0;
%             min_distance = 1e10;
%             for j = 1:length(path_x)
%                 distance = (x_set(i)-path_x(j))^2 + (y_set(i)-path_y(j))^2;
%                 if (min_distance > distance)
%                     min_distance = distance;
%                     init_search_index_set(i)=j;
%                     increase_count = 0;
%                 else
%                     increase_count = increase_count + 1;
%                 end
%                 if increase_count > 50
%                     break;
%                 end
%             end
%             match_point_index = init_search_index_set(i);
%             match_point_index_set(i) = match_point_index;
%             vector_match_point = [path_x(match_point_index);path_y(match_point_index)];
%             vector_match_point_direction = [cos(path_heading(match_point_index));sin(path_heading(match_point_index))];
%             vector_host_point = [x_set(i);y_set(i)];
%             vector_d = vector_host_point - vector_match_point;
%             vector_err = (vector_d'* vector_match_point_direction) * vector_match_point_direction;
%             vector_proj = vector_err + vector_match_point;
%             proj_x_set(i) = vector_proj(1);
%             proj_y_set(i) = vector_proj(2);
%             proj_heading_set(i) = path_heading(match_point_index) + path_kappa(match_point_index) * (vector_d'* vector_match_point_direction);
%             proj_kappa_set(i) = path_kappa(match_point_index);            
%         end
%     end 
% else
%     min_distance = inf;
%     for i = 1:length(x_set)
%         if isnan(x_set(i))
%             break;
%         else
%             increase_count = 0;
%             start_index = init_search_index_set(i);
%             vector_m_init = [path_x(start_index);path_y(start_index)];
%             vector_direction_init = [cos(path_heading(start_index));sin(path_heading(start_index))];
%             ds = ([x_set(1);y_set(1)]-vector_m_init)'*vector_direction_init;
%             if ds > 0            
%                 for j = start_index:length(path_x)
%                     distance = (x_set(i)-path_x(j))^2 + (y_set(i)-path_y(j))^2;
%                     if (min_distance > distance)
%                         min_distance = distance;
%                         init_search_index_set(i)=j;
%                         increase_count = 0;
%                     else
%                         increase_count = increase_count + 1;
%                     end
%                     if increase_count > 3
%                         break;
%                     end
%                 end
%             else
%                 for j = start_index:-1:1
%                     distance = (x_set(i)-path_x(j))^2 + (y_set(i)-path_y(j))^2;
%                     if (min_distance > distance)
%                         min_distance = distance;
%                         init_search_index_set(i)=j;
%                         increase_count = 0;
%                     else
%                         increase_count = increase_count + 1;
%                     end
%                     if increase_count > 3
%                         break;
%                     end
%                 end
%             end
%             match_point_index = init_search_index_set(i);
%             match_point_index_set(i) = match_point_index;
%             vector_match_point = [path_x(match_point_index);path_y(match_point_index)];
%             vector_match_point_direction = [cos(path_heading(match_point_index));sin(path_heading(match_point_index))];
%             vector_host_point = [x_set(i);y_set(i)];
%             vector_d = vector_host_point - vector_match_point;
%             vector_err = (vector_d'* vector_match_point_direction) * vector_match_point_direction;
%             vector_proj = vector_err + vector_match_point;
%             proj_x_set(i) = vector_proj(1);
%             proj_y_set(i) = vector_proj(2);
%             proj_heading_set(i) = path_heading(match_point_index) + path_kappa(match_point_index) * (vector_d'* vector_match_point_direction);
%             proj_kappa_set(i) = path_kappa(match_point_index);            
%         end
%     end    
% end

function [match_point_index_set,proj_x_set,proj_y_set,proj_heading_set,proj_kappa_set] = fcn(x_set,y_set,path_x,path_y,path_heading,path_kappa)
%该函数是一个通用函数，找到x_set,y_set在path_x,path_y的匹配点的编号，以及投影点在直角坐标系下的(x,y,theta,kappa)
%最多可以处理128个点

match_point_index_set = ones(128,1)*nan;
proj_x_set = ones(128,1)*nan;
proj_y_set = ones(128,1)*nan;
proj_heading_set = ones(128,1)*nan;
proj_kappa_set = ones(128,1)*nan;


persistent is_first_run;
persistent init_search_index_set;
if isempty(is_first_run)
    is_first_run = 0; 
    init_search_index_set = ones(128,1)*nan;
    for i = 1:length(x_set)
        if isnan(x_set(i))
            break;
        else
            increase_count = 0;
            min_distance = 1e10;
            for j = 1:length(path_x)
                distance = (x_set(i)-path_x(j))^2 + (y_set(i)-path_y(j))^2;
                if (min_distance > distance)
                    min_distance = distance;
                    init_search_index_set(i)=j;
                    increase_count = 0;
                else
                    increase_count = increase_count + 1;
                end
                if increase_count > 50
                    break;
                end
            end
            match_point_index = init_search_index_set(i);
            match_point_index_set(i) = match_point_index;
            vector_match_point = [path_x(match_point_index);path_y(match_point_index)];
            vector_match_point_direction = [cos(path_heading(match_point_index));sin(path_heading(match_point_index))];
            vector_host_point = [x_set(i);y_set(i)];
            vector_d = vector_host_point - vector_match_point;
            vector_err = (vector_d'* vector_match_point_direction) * vector_match_point_direction;
            vector_proj = vector_err + vector_match_point;
            proj_x_set(i) = vector_proj(1);
            proj_y_set(i) = vector_proj(2);
            proj_heading_set(i) = path_heading(match_point_index) + path_kappa(match_point_index) * (vector_d'* vector_match_point_direction);
            proj_kappa_set(i) = path_kappa(match_point_index);            
        end
    end 
else
    min_distance = inf;
    for i = 1:length(x_set)
        if isnan(x_set(i))
            break;
        else
            increase_count = 0;
            start_index = init_search_index_set(i);
            vector_m_init = [path_x(start_index);path_y(start_index)];
            vector_direction_init = [cos(path_heading(start_index));sin(path_heading(start_index))];
            ds = ([x_set(1);y_set(1)]-vector_m_init)'*vector_direction_init;

            if ds > 0            
                for j = start_index:length(path_x)
                    distance = (x_set(i)-path_x(j))^2 + (y_set(i)-path_y(j))^2;
                    if (min_distance > distance)
                        min_distance = distance;
                        init_search_index_set(i)=j;
                        increase_count = 0;
                    else
                        increase_count = increase_count + 1;
                    end
                    if increase_count > 3
                        break;
                    end
                end
            else
                for j = start_index:-1:1
                    distance = (x_set(i)-path_x(j))^2 + (y_set(i)-path_y(j))^2;
                    if (min_distance > distance)
                        min_distance = distance;
                        init_search_index_set(i)=j;
                        increase_count = 0;
                    else
                        increase_count = increase_count + 1;
                    end
                    if increase_count > 3
                        break;
                    end
                end
            end
            match_point_index = init_search_index_set(i);
            match_point_index_set(i) = match_point_index;
            vector_match_point = [path_x(match_point_index);path_y(match_point_index)];
            vector_match_point_direction = [cos(path_heading(match_point_index));sin(path_heading(match_point_index))];
            vector_host_point = [x_set(i);y_set(i)];
            vector_d = vector_host_point - vector_match_point;
            vector_err = (vector_d'* vector_match_point_direction) * vector_match_point_direction;
            vector_proj = vector_err + vector_match_point;
            proj_x_set(i) = vector_proj(1);
            proj_y_set(i) = vector_proj(2);
            proj_heading_set(i) = path_heading(match_point_index) + path_kappa(match_point_index) * (vector_d'* vector_match_point_direction);
            proj_kappa_set(i) = path_kappa(match_point_index);            
        end
    end    
end
%    if ds > 0            
%                 for j = start_index:length(path_x)
%                     distance = (x_set(i)-path_x(j))^2 + (y_set(i)-path_y(j))^2;
%                     if (min_distance > distance)
%                         min_distance = distance;
%                         init_search_index_set(i)=j;
%                         increase_count = 0;
%                     else
%                         increase_count = increase_count + 1;
%                     end
%                     if increase_count > 3
%                         break;
%                     end
%                 end
% else
%                 for j = start_index:-1:1
%                     distance = (x_set(i)-path_x(j))^2 + (y_set(i)-path_y(j))^2;
%                     if (min_distance > distance)
%                         min_distance = distance;
%                         init_search_index_set(i)=j;
%                         increase_count = 0;
%                     else
%                         increase_count = increase_count + 1;
%                     end
%                     if increase_count > 3
%                         break;
%                     end
%                 end
%             end
%             match_point_index = init_search_index_set(i);
%             match_point_index_set(i) = match_point_index;
%             vector_match_point = [path_x(match_point_index);path_y(match_point_index)];
%             vector_match_point_direction = [cos(path_heading(match_point_index));sin(path_heading(match_point_index))];
%             vector_host_point = [x_set(i);y_set(i)];
%             vector_d = vector_host_point - vector_match_point;
%             vector_err = (vector_d'* vector_match_point_direction) * vector_match_point_direction;
%             vector_proj = vector_err + vector_match_point;
%             proj_x_set(i) = vector_proj(1);
%             proj_y_set(i) = vector_proj(2);
%             proj_heading_set(i) = path_heading(match_point_index) + path_kappa(match_point_index) * (vector_d'* vector_match_point_direction);
%             proj_kappa_set(i) = path_kappa(match_point_index);            
%         end
%     end    
% end
% 
% 
% 
% 
%

== matlab function testemplanner_cs_old/Audi_A8_Sedan_1/Perciption/Perception Model ==
  data: host_x input; obs_x_set_gcs output; host_y input; host_heading_xy input; obs_range input; obs_theta input; obs_velocity input; obs_heading input; obs_y_set_gcs output; obs_velocity_set_gcs output; obs_heading_set_gcs output
function [obs_x_set_gcs,obs_y_set_gcs,obs_velocity_set_gcs,obs_heading_set_gcs] = fcn(host_x,host_y,host_heading_xy,obs_range,obs_theta,obs_velocity,obs_heading)

%作用：处理传感器所得到的障碍物信息，将其转换为世界坐标系下的障碍物信息。AIR传感器探测到的障碍物速度为世界坐标系下的绝对速度，距离为车辆坐标系下的相对距离，而航向则是以正北为正方向，顺时针为正，
%世界坐标系则是以正东为正方向，逆时针为正，因此需要进行变换(Heading [degs]: Compass heading of the target detected (driving direction where N = 0 degs, E = 90 degs, S = 180 degs and W = 270 degs))
%输入：车辆当前x,y位置和航向
%输出：障碍物在世界坐标系下的x,y位置、速度和航向     
obs_x_set_gcs=ones(32,1)*nan;
obs_y_set_gcs=ones(32,1)*nan;
obs_velocity_set_gcs=ones(32,1)*nan;
obs_heading_set_gcs=ones(32,1)*nan;
%传感器的极坐标航向角顺时针为正，世界坐标系下逆时针为正，需要做一个变换
theta_transfer=-obs_theta/180*pi;
%heading方向从正北为0变换为正东为0，同时顺时针和逆时针要变换
heading_transfer=-(obs_heading-90*ones(32,1))/180*pi;

for i=1:32
    if obs_range(i)~=0
        obs_x_set_gcs(i)=host_x+obs_range(i)*cos(host_heading_xy+theta_transfer(i))+3.8*cos(host_heading_xy);%x坐标分为三部分，①车辆的x坐标，②传感器和障碍物在世界坐标系下的x距离，③传感器与车辆坐标原点（后轴中心）的x方向距离
        obs_y_set_gcs(i)=host_y+obs_range(i)*sin(host_heading_xy+theta_transfer(i))+3.8*sin(host_heading_xy);%y坐标的组成与x坐标一致
        obs_velocity_set_gcs(i)=obs_velocity(i);%速度是绝对速度
        obs_heading_set_gcs(i)=heading_transfer(i);%航向角是转换后的航向角
    else
        
    end
    
end
end
